simulink model "self_balance_cart"  (R2021a)
settings: Solver=VariableStepAuto  StartTime=0.0  StopTime=20  RelTol=1e-3
values from neighbouring files (symbols this model uses):
  K = lqr(A,B,Q,R)    [lqr_self_balancing_robot.m]
settings Model: Creator=Admin  LastModifiedBy=Admin

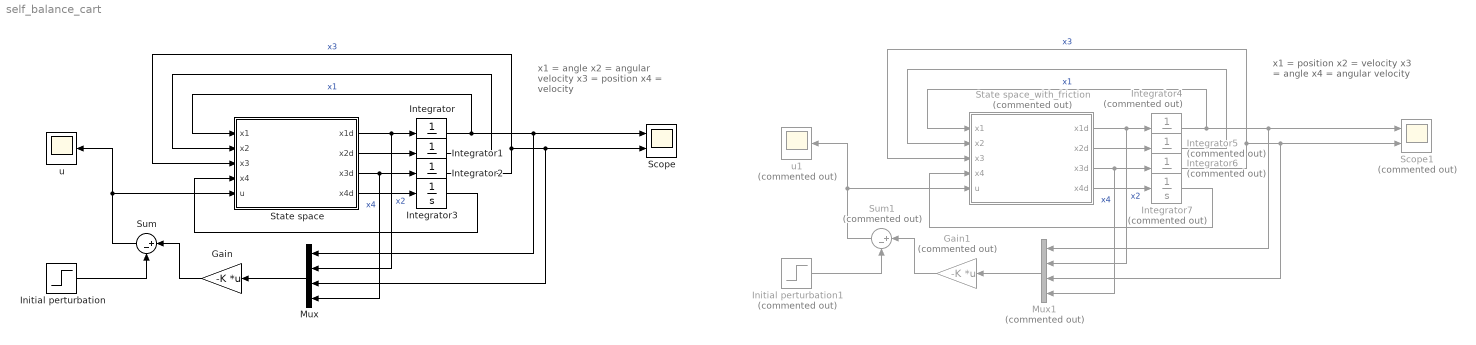
== system self_balance_cart ==
  note: x1 = angle
      | x2 = angular velocity
      | x3 = position
      | x4 = velocity
  note: x1 = position
      | x2 = velocity
      | x3 = angle
      | x4 = angular velocity
  Gain : Gain  Gain=-K  Multiplication=Matrix(K*u)
  Gain1 : Gain  Commented=on  Gain=-K  Multiplication=Matrix(K*u)
  Initial perturbation : Step  Time=0.01  Before=0.2  After=0  SampleTime=0
  Initial perturbation1 : Step  Commented=on  Time=0.01  Before=10  After=0  SampleTime=0
  Integrator{,1..3} (4 alike) : Integrator
  Integrator{4..7} (4 alike) : Integrator  Commented=on
  Mux : Mux
  Mux1 : Mux  Commented=on
  Scope : Scope  NumInputPorts=2
  Scope1 : Scope  Commented=on  NumInputPorts=2
  State space : MATLAB Function  TreatAsAtomicUnit=on
  State space_with_friction : MATLAB Function  Commented=on  TreatAsAtomicUnit=on
  Sum : Sum  Inputs=|+-
  Sum1 : Sum  Commented=on  Inputs=|+-
  u : Scope
  u1 : Scope  Commented=on
  wires:
  State space/1(x1d) -> Mux/2, Integrator/1  "x2"
  State space/2(x2d) -> Integrator1/1
  State space/3(x3d) -> Mux/4, Integrator2/1  "x4"
  State space/4(x4d) -> Integrator3/1
  Integrator/1 -> State space/1(x1), Mux/1, Scope/1  "x1"
  Integrator1/1 -> State space/2(x2)
  Integrator2/1 -> State space/3(x3), Mux/3, Scope/2  "x3"
  Integrator3/1 -> State space/4(x4)
  Mux/1 -> Gain/1
  Gain/1 -> Sum/1
  Sum/1 -> State space/5(u), u/1
  Initial perturbation/1 -> Sum/2
  State space_with_friction/1(x1d) -> Mux1/2, Integrator4/1  "x2"
  Mux1/1 -> Gain1/1
  Gain1/1 -> Sum1/1
  State space_with_friction/4(x4d) -> Integrator7/1
  Sum1/1 -> State space_with_friction/5(u), u1/1
  Integrator5/1 -> State space_with_friction/2(x2)
  Integrator7/1 -> State space_with_friction/4(x4)
  Initial perturbation1/1 -> Sum1/2
  Integrator4/1 -> State space_with_friction/1(x1), Scope1/1, Mux1/1  "x1"
  State space_with_friction/3(x3d) -> Mux1/4, Integrator6/1  "x4"
  Integrator6/1 -> State space_with_friction/3(x3), Scope1/2, Mux1/3  "x3"
  State space_with_friction/2(x2d) -> Integrator5/1

== matlab function self_balance_cart/State space_with_friction ==
  data: x1 input; x2 input; x3 input; x4 input; u input; x1d output; x2d output; x3d output; x4d output
function [x1d,x2d,x3d,x4d] = fcn(x1,x2,x3,x4,u)
m = 1.177;
M = 0.192;
l = 0.05;
I = 0.0029;
g = 9.81;
b = 0.1;
r = 0.04;

p = (M+m)*I+M*m*l^2;  %denominator for the A and B matrices
A1 = -(I+M*l^2)*b/p;
A2 = (M^2*g*l^2)/p;
A3 = -(M*l*b)/p;
A4 = M*g*l*(M+m)/p;
B1 = (I+M*l^2)/p;
B2 = m*l/p;

x1d = x2;
x2d = A1*x2+A2*x3+B1*u;
x3d = x4;
x4d = A3*x2+A4*x3+B2*u; 


% A = [0      1              0           0;
%      0      A1             A2          0;
%      0      0              0           1;
%      0      A3             A4          0];
% B =      [0;
%           B1;
%           0;
%           B2];
% C = [1 0 0 0;
%      0 0 1 0];
% D = [0;
%      0];
% 
% 
% Q = [200   0     0     0
%      0     0     0     0
%      0     0    150    0
%      0     0     0     0]
%  
% R = 1;
% 
% K = lqr(A,B,Q,R)

== matlab function self_balance_cart/State space ==
  data: x1 input; x2 input; x3 input; x4 input; u input; x1d output; x2d output; x3d output; x4d output
function [x1d,x2d,x3d,x4d] = fcn(x1,x2,x3,x4,u)
m = 1.177;
M = 0.192;
l = 0.05;
I = 0.0029;
g = 9.81;
r = 0.04;

A1 = ((M+m)*m*g*l)/((M+m)*I+M*m*l^2);
B1 = (m*l)/((M+m)*I+M*m*l^2);
A2 = ((m^2)*g*l^2)/((M+m)*I+M*m*l^2);
B2 = (I+m*l^2)/((M+m)*I+M*m*l^2);

x1d = x2;
x2d = A1*x1-B1*u;
x3d = x4;
x4d = -A2*x1+B2*u; 

% A = [0      1              0           0;
%      A1     0              0           0;
%      0      0              0           1;
%     -A2     0              0           0];
% B =      [0;
%          -B1;
%           0;
%           B2];
% C = [1 0 0 0;
%      0 0 1 0];
% D = [0;
%      0];
% 
% 
% Q = [200   0     0     0
%      0     0     0     0
%      0     0    150    0
%      0     0     0     0]
%  
% R = 1;
% 
% K = lqr(A,B,Q,R)
